simulink model "sampleModel1671_2_sub_sub"  (R2023a)
settings: Solver=VariableStepAuto  StartTime=0.0  StopTime=10.0  RelTol=1e-3
libraries: hdlsllib x5, simulink x1
settings Model: Creator=user1  LastModifiedBy=user1
settings OptimizationCC: BlockReduction=off  ConditionallyExecuteInputs=off

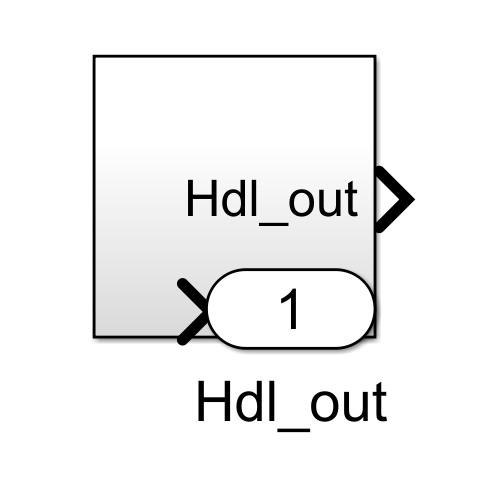
[thumbnail: Simulink's stored preview of the top-level diagram]
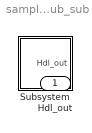
== system sampleModel1671_2_sub_sub ==
  Subsystem : Subsystem
  Hdl_out : Outport  OutDataTypeStr=uint8

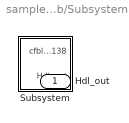
== system sampleModel1671_2_sub_sub/Subsystem ==
  Subsystem : Subsystem
  Hdl_out : Outport  OutDataTypeStr=uint8

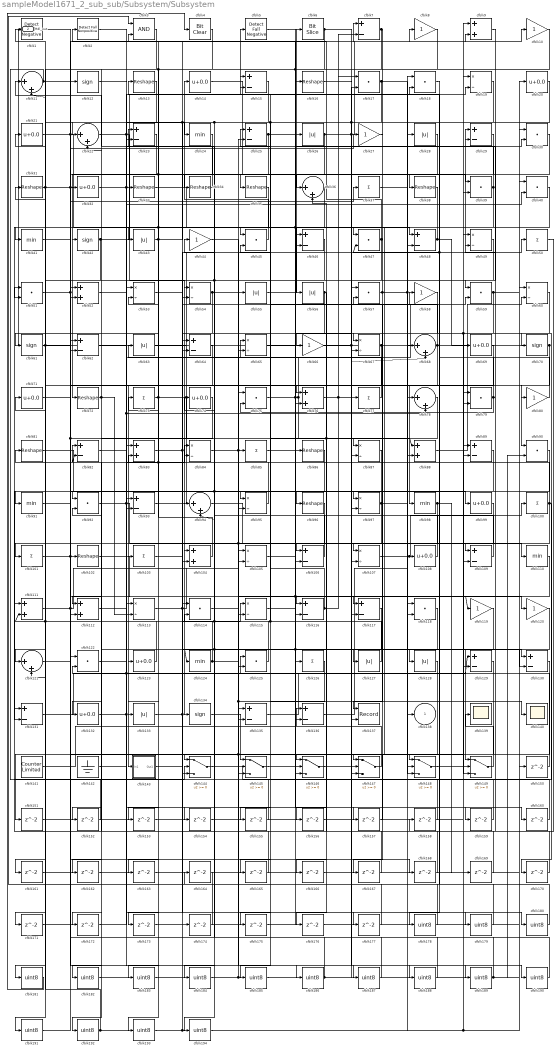
== system sampleModel1671_2_sub_sub/Subsystem/Subsystem ==
  cfblk1 : hdlsllib/Logic and Bit Operations/Detect Fall Negative  vinit=0  OutDataTypeStr=uint8
  cfblk{8,10,27,44,58,66,80,119..120} (9 alike) : Gain  OutDataTypeStr=uint8
  cfblk{37,50,73,77,85,100..101,103,126} (9 alike) : Sum  Inputs=+  OutDataTypeStr=uint8
  cfblk{13,16,31,33..35,38,72,81,86,96,102} (12 alike) : Reshape
  cfblk{9,52,76,83,88,104,111..112} (8 alike) : Sum  OutDataTypeStr=uint8
  cfblk{19,49,53..54,60,65,67,84,87,95,97,105,107,113,115} (15 alike) : Product  Inputs=*/  OutDataTypeStr=uint8  RndMeth=Zero  SaturateOnIntegerOverflow=on
  cfblk{7,15,23,25,29,46,48,62,64,82,89,93,106,109,116..117,129..131,135..136} (21 alike) : Sum  Inputs=+-  OutDataTypeStr=uint8
  cfblk{14,20..21,32,69,71,74,99,108,123,132} (11 alike) : Bias  Bias=0.0  SaturateOnIntegerOverflow=off
  cfblk{11,22,36,68,78,94,121} (7 alike) : Sum  Inputs=|++  OutDataTypeStr=uint8
  cfblk{24,41,91,98,110,124} (6 alike) : MinMax  OutDataTypeStr=uint8
  cfblk{17..18,30,39..40,45,47,51,57,59,75,79,90,92,114,118,122,125} (18 alike) : DotProduct  OutDataTypeStr=uint8
  cfblk{12,42,61,70,134} (5 alike) : Signum
  cfblk{26,28,43,55..56,63,127..128,133} (9 alike) : Abs  OutDataTypeStr=uint8  SaturateOnIntegerOverflow=off
  cfblk137 : Record  FileSettingsInternal="{\"entries\":[{\"content\":{\"excelSettings\":{\"content\":{},\"type\":\"Streamout.ExcelSettings\"}},\"type\":\"Streamout.FileSettingStorage\",\"uuid\":\"\"}],\"packageUris\":[\"http:\\/\\/schema.mathworks.com\\/mf0\\/streamout_blocks\\/R2020a\"],\"version\":\"1.0\"}"  Layout=[1 1]  SignalsInternal="{\"entries\":[{\"content\":{\"signals\":[{\"content\":{\"blockPath\":[],\"dimensions\":[1],\"domain\":\"\",\"lineColor\":\"#a2142f\",\"plots\":[1],\"port\":1,\"signalID\":33257,\"signalName\":\"cfblk58\"},\"type\":\"RecordBlkView.Signal\",\"uuid\":\"\"},{\"content\":{\"blockPath\":[],\"dimensions\":[1],\"domain\":\"\",\"lineColor\":\"#139fff\",\"plots\":[1],\"port\":2,\"signalID\":33260,\"signalName\":\"cfblk81\"},\"type\":\"RecordBlkView.Signal\",\"uuid\":\"\"}]},\"type\":\"RecordBlkView.InputSignals\",\"uuid\":\"\"}],\"packageUris\":[\"http:\\/\\/schema.mathworks.com\\/mf0\\/streamout_blocks\\/R2020a\"],\"version\":\"1.0\"}"  VisualizationBindings="{\"xyplotplugin\":{\"info\":[{\"series\":[{\"bindingParametersList\":[{\"parameter\":\"X-Axis\",\"signalID\":33257,\"signalName\":\"cfblk58\"},{\"parameter\":\"Y-Axis\",\"signalID\":33260,\"signalName\":\"cfblk81\"}],\"seriesID\":62957}],\"subplotID\":1}]}}"  CompatibilityTag=XY  st=-1
  cfblk139 : Scope
  cfblk140 : Scope
  cfblk141 : hdlsllib/Sources/Counter Limited  uplimit=7  tsamp=-1
  cfblk142 : Ground
  cfblk143 : Subsystem
      settings: LibrarySourceBlock=|
      | hdlsllib/Ports &
      | Subsystems/Subsystem
  cfblk{144..149} (6 alike) : Switch  OutDataTypeStr=uint8  SaturateOnIntegerOverflow=off  InputSameDT=off
  cfblk{150..177} (28 alike) : Delay  SampleTime=1
  cfblk{178..194} (17 alike) : DataTypeConversion  OutDataTypeStr=uint8  SaturateOnIntegerOverflow=off  RndMeth=Floor
  cfblk2 : hdlsllib/Logic and Bit Operations/Detect Fall Nonpositive  vinit=0  OutDataTypeStr=uint8
  cfblk3 : Logic  AllPortsSameDT=off  OutDataTypeStr=boolean
  cfblk4 : simulink/Logic and Bit Operations/Bit Clear  iBit=0
      settings: LibrarySourceBlock=|
      | hdlsllib/Logic and Bit
      | Operations/Bit Clear
  cfblk5 : hdlsllib/Logic and Bit Operations/Detect Fall Negative  vinit=0  OutDataTypeStr=uint8
  cfblk6 : hdlsllib/Logic and Bit Operations/Bit Slice  lidx=7  ridx=0
  cfblk138 : Outport  OutDataTypeStr=uint8  VectorParamsAs1DForOutWhenUnconnected=off
  Hdl_out : Outport  Port=2  OutDataTypeStr=uint8
  wires:
  cfblk194/1 -> cfblk118/2
  cfblk193/1 -> cfblk118/1
  cfblk24/1 -> cfblk193/1
  cfblk192/1 -> cfblk20/1, cfblk109/2, cfblk174/1, cfblk31/1
  cfblk191/1 -> cfblk52/2
  cfblk3/1 -> cfblk191/1
  cfblk190/1 -> cfblk52/1
  cfblk16/1 -> cfblk190/1
  cfblk189/1 -> cfblk164/1, cfblk90/2
  cfblk188/1 -> cfblk114/2
  cfblk176/1 -> cfblk188/1
  cfblk187/1 -> cfblk114/1
  cfblk186/1 -> cfblk39/2, cfblk122/1
  cfblk185/1 -> cfblk89/2
  cfblk117/1 -> cfblk185/1
  cfblk184/1 -> cfblk89/1
  cfblk183/1 -> cfblk150/1
  cfblk89/1 -> cfblk183/1
  cfblk182/1 -> cfblk17/2, cfblk105/2
  cfblk181/1 -> cfblk4/1
  cfblk87/1 -> cfblk181/1
  cfblk180/1 -> cfblk18/2
  cfblk179/1 -> cfblk18/1
  cfblk2/1 -> cfblk179/1
  cfblk178/1 -> cfblk53/1
  cfblk18/1 -> cfblk178/1
  cfblk177/1 -> cfblk1/1
  cfblk175/1 -> cfblk60/1
  cfblk174/1 -> cfblk62/1
  cfblk173/1 -> cfblk46/2
  cfblk172/1 -> cfblk83/1
  cfblk171/1 -> cfblk23/2
  cfblk170/1 -> cfblk29/2
  cfblk169/1 -> cfblk36/2
  cfblk168/1 -> cfblk111/1
  cfblk167/1 -> cfblk64/1
  cfblk130/1 -> cfblk167/1
  cfblk166/1 -> cfblk48/2
  cfblk128/1 -> cfblk166/1
  cfblk165/1 -> cfblk92/2
  cfblk126/1 -> cfblk165/1
  cfblk164/1 -> cfblk3/1
  cfblk163/1 -> cfblk135/1
  cfblk162/1 -> cfblk93/1
  cfblk74/1 -> cfblk162/1
  cfblk161/1 -> cfblk40/1
  cfblk160/1 -> cfblk105/1
  cfblk159/1 -> cfblk75/1
  cfblk158/1 -> cfblk51/1
  cfblk50/1 -> cfblk158/1
  cfblk157/1 -> cfblk57/2
  cfblk145/1 -> cfblk157/1
  cfblk156/1 -> cfblk68/1
  cfblk155/1 -> cfblk84/2
  cfblk154/1 -> cfblk88/2
  cfblk112/1 -> cfblk154/1
  cfblk153/1 -> cfblk79/2
  cfblk152/1 -> cfblk131/1
  cfblk151/1 -> cfblk25/2
  cfblk129/1 -> cfblk151/1
  cfblk150/1 -> cfblk122/2
  cfblk13/1 -> cfblk41/1
  cfblk148/1 -> cfblk100/1
  cfblk38/1 -> cfblk112/2, cfblk153/1
  cfblk37/1 -> cfblk129/2
  cfblk67/1 -> cfblk121/1, cfblk117/1
  cfblk143/1(Out1) -> cfblk125/1
  cfblk81/1 -> cfblk137/2
  cfblk104/1 -> cfblk83/2
  cfblk83/1 -> cfblk46/1, cfblk127/1
  cfblk91/1 -> cfblk37/1
  cfblk103/1 -> cfblk59/2
  cfblk29/1 -> cfblk32/1
  cfblk105/1 -> cfblk10/1
  cfblk61/1 -> cfblk117/2, cfblk161/1
  cfblk82/1 -> cfblk65/1
  cfblk99/1 -> cfblk104/2, cfblk125/2
  cfblk36/1 -> cfblk124/1, cfblk194/1
  cfblk52/1 -> cfblk189/1
  cfblk101/1 -> cfblk8/1, cfblk168/1
  cfblk62/1 -> cfblk33/1, cfblk30/2
  cfblk95/1 -> cfblk73/1, cfblk82/2
  cfblk121/1 -> cfblk146/1
  cfblk149/1 -> cfblk139/1
  cfblk131/1 -> cfblk79/1
  cfblk44/1 -> cfblk147/1
  cfblk147/1 -> cfblk136/1
  cfblk73/1 -> cfblk115/2, cfblk9/1, cfblk3/2
  cfblk57/1 -> cfblk28/1, cfblk149/3, cfblk87/1
  cfblk71/1 -> cfblk145/2, cfblk87/2
  cfblk78/1 -> cfblk155/1, cfblk156/1
  cfblk31/1 -> cfblk113/1, cfblk39/1, cfblk171/1
  cfblk110/1 -> cfblk135/2
  cfblk134/1 -> cfblk145/1
  cfblk54/1 -> cfblk140/1, cfblk64/2
  cfblk85/1 -> cfblk86/1
  cfblk116/1 -> cfblk45/2, cfblk7/2
  cfblk58/1 -> cfblk137/1
  cfblk122/1 -> cfblk84/1
  cfblk68/1 -> cfblk25/1, cfblk112/1
  cfblk142/1 -> cfblk129/1, cfblk19/2
  cfblk75/1 -> cfblk49/1, cfblk107/2, cfblk80/1
  cfblk141/1 -> cfblk116/2
  cfblk25/1 -> cfblk93/2, cfblk99/1
  cfblk26/1 -> cfblk172/1, cfblk173/1, cfblk9/2, cfblk148/1
  cfblk120/1 -> cfblk149/1
  cfblk8/1 -> cfblk22/1
  cfblk136/1 -> cfblk78/1
  cfblk53/1 -> cfblk97/2
  cfblk125/1 -> cfblk11/2, cfblk111/2, cfblk74/1
  cfblk9/1 -> cfblk59/1
  cfblk133/1 -> cfblk115/1, cfblk146/3
  cfblk21/1 -> cfblk48/1, cfblk34/1
  cfblk124/1 -> cfblk148/2, cfblk177/1, cfblk136/2, cfblk71/1
  cfblk40/1 -> cfblk54/2, cfblk76/2
  cfblk107/1 -> cfblk19/1, cfblk108/1
  cfblk27/1 -> cfblk107/1
  cfblk6/1 -> cfblk148/3, cfblk163/1
  cfblk115/1 -> cfblk106/2
  cfblk48/1 -> cfblk47/1, cfblk69/1
  cfblk15/1 -> cfblk54/1
  cfblk11/1 -> cfblk144/2, cfblk76/1
  cfblk30/1 -> cfblk42/1
  cfblk86/1 -> cfblk131/2, cfblk184/1
  cfblk17/1 -> cfblk94/2, cfblk43/1, cfblk138/1
  cfblk92/1 -> cfblk78/2, cfblk15/1, cfblk110/1
  cfblk35/1 -> cfblk51/2
  cfblk51/1 -> cfblk27/1, cfblk187/1
  cfblk72/1 -> cfblk92/1, cfblk113/2
  cfblk127/1 -> cfblk82/1, cfblk15/2
  cfblk12/1 -> cfblk24/1
  cfblk119/1 -> cfblk128/1
  cfblk77/1 -> cfblk63/1
  cfblk28/1 -> cfblk36/1
  cfblk66/1 -> cfblk58/1, cfblk68/2
  cfblk108/1 -> cfblk23/1
  cfblk123/1 -> cfblk21/1
  cfblk111/1 -> cfblk12/1, cfblk65/2
  cfblk113/1 -> cfblk55/1, cfblk180/1
  cfblk46/1 -> cfblk94/1, cfblk132/1
  cfblk1/1 -> cfblk88/1, cfblk95/1
  cfblk59/1 -> cfblk145/3, cfblk149/2, cfblk30/1
  cfblk102/1 -> cfblk116/1
  cfblk97/1 -> cfblk91/1, cfblk120/1, cfblk152/1
  cfblk88/1 -> cfblk60/2
  cfblk5/1 -> cfblk67/2
  cfblk84/1 -> cfblk85/1, cfblk130/1
  cfblk135/1 -> cfblk57/1
  cfblk41/1 -> cfblk102/1
  cfblk146/1 -> cfblk77/1
  cfblk10/1 -> cfblk133/1, cfblk62/2, cfblk146/2
  cfblk63/1 -> cfblk50/1
  cfblk19/1 -> cfblk45/1, cfblk147/2
  cfblk118/1 -> cfblk192/1
  cfblk65/1 -> cfblk126/1, cfblk130/2, cfblk119/1
  cfblk42/1 -> cfblk5/1, cfblk121/2
  cfblk60/1 -> cfblk66/1
  cfblk98/1 -> cfblk101/1, cfblk169/1
  cfblk56/1 -> cfblk104/1, cfblk176/1
  cfblk34/1 -> cfblk11/1
  cfblk23/1 -> cfblk72/1
  cfblk100/1 -> cfblk123/1, cfblk53/2, cfblk170/1
  cfblk22/1 -> cfblk134/1, cfblk147/3
  cfblk4/1 -> cfblk182/1
  cfblk20/1 -> cfblk144/3, cfblk22/2, cfblk175/1
  cfblk33/1 -> cfblk56/1
  cfblk109/1 -> cfblk81/1
  cfblk80/1 -> cfblk13/1, cfblk47/2
  cfblk32/1 -> cfblk35/1
  cfblk144/1 -> cfblk70/1
  cfblk93/1 -> cfblk29/1
  cfblk43/1 -> cfblk61/1, cfblk7/1
  cfblk14/1 -> cfblk38/1
  cfblk79/1 -> cfblk75/2, cfblk16/1, cfblk49/2
  cfblk76/1 -> cfblk17/1, cfblk160/1
  cfblk96/1 -> cfblk106/1
  cfblk90/1 -> cfblk96/1
  cfblk69/1 -> cfblk98/1
  cfblk94/1 -> cfblk109/1
  cfblk49/1 -> cfblk97/1
  cfblk45/1 -> cfblk14/1
  cfblk132/1 -> cfblk40/2, cfblk159/1
  cfblk114/1 -> cfblk186/1
  cfblk55/1 -> cfblk6/1
  cfblk106/1 -> cfblk44/1
  cfblk39/1 -> cfblk144/1, cfblk26/1
  cfblk7/1 -> cfblk67/1, cfblk103/1
  cfblk70/1 -> cfblk90/1, Hdl_out/1
  cfblk64/1 -> cfblk143/1(In1)
  cfblk47/1 -> cfblk2/1, cfblk95/2

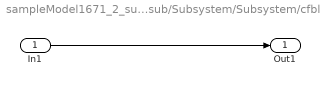
== system sampleModel1671_2_sub_sub/Subsystem/Subsystem/cfblk143 ==
  In1 : Inport
  Out1 : Outport
  wires:
  In1/1 -> Out1/1
